simulink model "FFM_Punch"  (R2017a)
settings: Solver=ode3  StartTime=0.0  StopTime=timesteps  FixedStep=data.SIM.Ts  RelTol=1e-3  EnableMultiTasking=on
values from neighbouring files (symbols this model uses):
  data =     [dakota_config.mat]
  downshift_map = data.TCU.upshift.veh_spd_default    [Simulation_results.m]
  upshift_map = data.TCU.upshift.veh_spd_default    [Simulation_results.m]
undefined symbols (not defined in the file or in its folder): air_density, Cd, DiscIntNeverNeededParam, fr_crankshaft, fr_speed_values, g, i_FD, ICE, Low_Ratio, M_Eng_Max, M_Eng_Max_Max, M_Eng_Max_Rpm, mt2m_f, mu_Roll_C0, mu_Roll_C1, mu_Roll_C2, Mv, n_Idle_Eng, Overdrive_Ratio, Re, S_eff_drag, Ts
(part 11 of 15)

== system FFM_Punch/Driver Interface/Driver Model-_old/Driver Pedal Behaviour/Saturation Dynamic1 ==
  up : Inport
  u : Inport  Port=2
  lo : Inport  Port=3
  Data Type Duplicate : DataTypeDuplicate  DisableCoverage=on
  Data Type Propagation : S-Function  FunctionName=sfix_dtprop  Parameters=14,PropDataTypeMode,(getdatatypespecs(PropDataType,PropScaling,DblOver,0, 0, PropDataTypeMode, PropScalingMode)),IfRefDouble,IfRefSingle,IsSigned,NumBitsBase,NumBitsMult,NumBitsAdd,(sort(reshape(round(NumBitsAllowFinal), prod(size(NumBitsAllowFinal)),1))),PropScalingMode,ValuesUsedBestPrec,SlopeBase,SlopeMult,SlopeAdd,BiasBase,BiasMult,BiasAdd,DblOver  SFunctionDeploymentMode=off  EnableBusSupport=off  mask(Data Type Propagation){PropDataTypeMode=Inherit via propagation rule, PropDataType=fixdt(1, 16), IfRefDouble=double, IfRefSingle=single, IsSigned=IsSigned1, NumBitsBase=NumBits1, NumBitsMult=1, NumBitsAdd=0, NumBitsAllowFinal=1:128, PropScalingMode=Inherit via propagation rule, PropScaling=2^-10, ValuesUsedBestPrec=[5 -7], SlopeBase=Slope1, SlopeMult=1, SlopeAdd=0, BiasBase=Bias1, BiasMult=1, BiasAdd=0}
      mask prompts: PropDataTypeMode "Simulink:masks:x1PropagatedDataType_MP"; PropDataType "Simulink:masks:x11PropagatedDataTypeegFixdt116Fixdtsingle_MP"; IfRefDouble "Simulink:masks:x11IfAnyReferenceInputIsDoubleOutputIs_MP"; IfRefSingle "Simulink:masks:x12IfAnyReferenceInputIsSingleOutputIs_MP"; IsSigned "Simulink:masks:x13IsSigned_MP"; NumBitsBase "Simulink:masks:x141NumberofBitsBase_MP"; NumBitsMult "Simulink:masks:x142NumberofBitsMultiplicativeAdjustment_MP"; NumBitsAdd "Simulink:masks:x143NumberofBitsAdditiveAdjustment_MP"; NumBitsAllowFinal "Simulink:masks:x144NumberofBitsAllowableFinalValues_MP"; PropScalingMode "Simulink:masks:x2PropagatedScaling_MP"; PropScaling "Simulink:masks:x21PropagatedScalingSlopeEg29OrSlopeBiasEg1253_MP"; ValuesUsedBestPrec "Simulink:masks:x21ValuesUsedToDetermineBestPrecisionScaling_MP"; SlopeBase "Simulink:masks:x211SlopeBase_MP"; SlopeMult "Simulink:masks:x212SlopeMultiplicativeAdjustment_MP"; SlopeAdd "Simulink:masks:x213SlopeAdditiveAdjustment_MP"; BiasBase "Simulink:masks:x221BiasBase_MP"; BiasMult "Simulink:masks:x222BiasMultiplicativeAdjustment_MP"; BiasAdd "Simulink:masks:x223BiasAdditiveAdjustment_MP"
      mask help: Simulink:masks:DataTypePropagation_MD
      mask init:
      | DblOver = 0;
      mask TypeOptions PropDataTypeMode: Simulink:masks:SpecifyViaDialog | Simulink:masks:InheritViaPropagationRule
      mask Callback PropDataTypeMode: fixptdialog(gcbh)
      mask Callback PropDataType: fixptdialog(gcbh)
      mask TypeOptions IfRefDouble: Simulink:masks:double | Simulink:masks:single
      mask TypeOptions IfRefSingle: Simulink:masks:double | Simulink:masks:single
      mask TypeOptions IsSigned: Simulink:masks:IsSigned1 | Simulink:masks:IsSigned2 | Simulink:masks:IsSigned1OrIsSigned2 | Simulink:masks:TRUE | Simulink:masks:FALSE
      mask TypeOptions NumBitsBase: NumBits1 | NumBits2 | max([NumBits1 NumBits2]) | min([NumBits1 NumBits2]) | NumBits1+NumBits2
      mask TypeOptions PropScalingMode: Simulink:masks:SpecifyViaDialog | Simulink:masks:InheritViaPropagationRule | Simulink:masks:ObtainViaBestPrecision
      mask Callback PropScalingMode: fixptdialog(gcbh)
      mask TypeOptions SlopeBase: Slope1 | Slope2 | max([Slope1 Slope2]) | min([Slope1 Slope2]) | Slope1*Slope2 | Slope1/Slope2 | PosRange1 | PosRange2 | max([PosRange1 PosRange2]) | min([PosRange1 PosRange2]) | PosRange1*PosRange2 | PosRange1/PosRange2
      mask TypeOptions BiasBase: Bias1 | Bias2 | max([Bias1 Bias2]) | min([Bias1 Bias2]) | Bias1*Bias2 | Bias1/Bias2 | Bias1+Bias2 | Bias1-Bias2
      mask Display:
      | port_label('Input',1,'Ref1');
      | port_label('Input',2,'Ref2');
      | port_label('Input',3,'Prop');
  LowerRelop1 : RelationalOperator  DisableCoverage=on  Operator=>  OutDataTypeStr=boolean  RndMeth=Nearest
  Switch : Switch  Criteria=u2 ~= 0  OutDataTypeStr=Inherit: Inherit via back propagation  ZeroCross=off
  Switch2 : Switch  Criteria=u2 ~= 0  OutMin=OutMin  OutMax=OutMax  OutDataTypeStr=Inherit: Inherit via back propagation  ZeroCross=off
  UpperRelop : RelationalOperator  DisableCoverage=on  Operator=<  OutDataTypeStr=boolean  RndMeth=Nearest
  y : Outport  OutMin=OutMin  OutMax=OutMax
  wires:
  up/1 -> Switch2/1, LowerRelop1/2
  u/1 -> Data Type Propagation/2, Data Type Propagation/1, LowerRelop1/1, Switch/3, UpperRelop/1
  lo/1 -> Switch/1, UpperRelop/2
  Switch/1 -> Data Type Duplicate/2, Switch2/3, Data Type Propagation/3
  Switch2/1 -> Data Type Duplicate/1, y/1
  LowerRelop1/1 -> Switch2/2
  UpperRelop/1 -> Switch/2

== system FFM_Punch/Controller/F02_03_03_05_Raw_Gear_Target_Auto_Mode/F02_03_03_05_09_Final_Raw_Gear_Target_Auto_Mode/TurnOnDelay1/Rising_Edge_DetectChange1 ==
  b_Input : Inport  Tag=Controls_Lib  Description=Inp  OutDataTypeStr=boolean  Interpolate=off
  b_InitialValue : Inport  Tag=Controls_Lib  Description=Inp  Port=2  OutDataTypeStr=boolean  Interpolate=off
  Delay1 : Delay  Tag=Controls_Lib  Description=VariableDelay  DelayLength=DelayLength  DelayLengthUpperLimit=DelayLengthUpperLimit  InitialConditionSource=Input port  InitialCondition=InitialCondition  SampleTime=SampleTime  mask(Delay){DelayLengthSource=Dialog, DelayLength=1, DelayLengthUpperLimit=100, InitialConditionSource=Input port, InitialCondition=0.0, ExternalReset=None, PreventDirectFeedthrough=off, DiagnosticForOutOfRangeDelayLength=None, RemoveProtectionDelayLength=off, InputProcessing=Elements as channels (sample based), UseCircularBuffer=off, SampleTime=-1, StateName=, StateMustResolveToSignalObject=off, CodeGenStateStorageClass=Auto, CodeGenStateStorageTypeQualifier=}
      mask prompts: DelayLengthSource "Delay length source:"; DelayLength "Delay length:"; DelayLengthUpperLimit "Delay upper limit:"; InitialConditionSource "Initial condition source:"; InitialCondition "Initial condition:"; ExternalReset "External reset:"; PreventDirectFeedthrough "Prevent direct feedthrough by increasing delay length to lower limit"; DiagnosticForOutOfRangeDelayLength "Diagnostic for out-of-range delay length:"; RemoveProtectionDelayLength "Remove protection against out-of-range delay length in generated code"; InputProcessing "Input processing:"; UseCircularBuffer "Use circular buffer for state"; SampleTime "Sample time (-1 for inherited):"; StateName "State name:"; StateMustResolveToSignalObject "State name must resolve to Simulink signal object"; CodeGenStateStorageClass "Code generation storage class:"; CodeGenStateStorageTypeQualifier "Code generation storage type qualifier:"
      mask help: Delay input by a fixed or variable number of samples. The initial output of the delay block is specified by the external input x0.
      settings: InputPortMap=u0,p4
      mask Help: web([fileparts(which('Lib_discrete')) filesep 'hlp' filesep 'lib_Delay.html'], '-helpbrowser')
      mask TypeOptions DelayLengthSource: DelayLengthSource
      mask TypeOptions DelayLength: DelayLength
      mask TypeOptions DelayLengthUpperLimit: DelayLengthUpperLimit
      mask TypeOptions InitialConditionSource: InitialConditionSource
      mask TypeOptions InitialCondition: InitialCondition
      mask TypeOptions ExternalReset: ExternalReset
      mask TypeOptions PreventDirectFeedthrough: PreventDirectFeedthrough
      mask TypeOptions DiagnosticForOutOfRangeDelayLength: DiagnosticForOutOfRangeDelayLength
      mask TypeOptions RemoveProtectionDelayLength: RemoveProtectionDelayLength
      mask TypeOptions InputProcessing: InputProcessing
      mask TypeOptions UseCircularBuffer: UseCircularBuffer
      mask TypeOptions SampleTime: SampleTime
      mask TypeOptions StateName: StateName
      mask TypeOptions StateMustResolveToSignalObject: StateMustResolveToSignalObject
      mask TypeOptions CodeGenStateStorageClass: CodeGenStateStorageClass
      mask TypeOptions CodeGenStateStorageTypeQualifier: CodeGenStateStorageTypeQualifier
  Logic : Logic  Tag=Controls_Lib  Description=Logic  Operator=NOT  Inputs=Inputs  OutDataTypeStr=boolean  SampleTime=SampleTime  mask(Logic){Operator=NOT, Inputs=2, IconShape=rectangular, SampleTime=-1, AllPortsSameDT=on, OutDataTypeStr=boolean}
      mask prompts: Inputs "Number of input ports:"; IconShape "Icon shape:"; SampleTime "Sample time (-1 for inherited):"; AllPortsSameDT "Require all inputs and output to have the same data type"; OutDataTypeStr "Output data type:"
      mask help: Logical operators. For a single input, operators are applied across the input vector. For multiple inputs, operators are applied across the inputs.
      mask Help: web([fileparts(which('Lib_built')) filesep 'hlp' filesep 'lib_Logic' '.html'], '-helpbrowser')
      mask TypeOptions Operator: Operator
      mask TypeOptions Inputs: Inputs
      mask TypeOptions IconShape: IconShape
      mask TypeOptions SampleTime: SampleTime
      mask TypeOptions AllPortsSameDT: AllPortsSameDT
      mask TypeOptions OutDataTypeStr: OutDataTypeStr
  Logic1 : Logic  Tag=Controls_Lib  Description=Logic  Inputs=Inputs  OutDataTypeStr=boolean  SampleTime=SampleTime  mask(Logic){Operator=AND, Inputs=2, IconShape=rectangular, SampleTime=-1, AllPortsSameDT=on, OutDataTypeStr=boolean}
      mask prompts: Inputs "Number of input ports:"; IconShape "Icon shape:"; SampleTime "Sample time (-1 for inherited):"; AllPortsSameDT "Require all inputs and output to have the same data type"; OutDataTypeStr "Output data type:"
      mask help: Logical operators. For a single input, operators are applied across the input vector. For multiple inputs, operators are applied across the inputs.
      mask Help: web([fileparts(which('Lib_built')) filesep 'hlp' filesep 'lib_Logic' '.html'], '-helpbrowser')
      mask TypeOptions Operator: Operator
      mask TypeOptions Inputs: Inputs
      mask TypeOptions IconShape: IconShape
      mask TypeOptions SampleTime: SampleTime
      mask TypeOptions AllPortsSameDT: AllPortsSameDT
      mask TypeOptions OutDataTypeStr: OutDataTypeStr
  b_Output : Outport  Tag=Controls_Lib  OutDataTypeStr=boolean
  wires:
  Delay1/1 -> Logic/1
  Logic1/1 -> b_Output/1
  Logic/1 -> Logic1/2
  b_Input/1 -> Logic1/1, Delay1/1
  b_InitialValue/1 -> Delay1/2

== system FFM_Punch/Controller/F02_03_03_05_Raw_Gear_Target_Auto_Mode/F02_03_03_05_09_Final_Raw_Gear_Target_Auto_Mode/TurnOnDelay1/Timer ==
  note: Reset check
  Res : Inport  Tag=Controls_Lib_V1.0  OutDataTypeStr=boolean  Interpolate=off
  TT : Inport  Tag=Controls_Lib_V1.0  Port=2  OutDataTypeStr=single  Interpolate=off
  AddSub1 : Sum  Tag=Controls_Lib  Description=AddSub  Inputs=-+  CollapseDim=CollapseDim  AccumDataTypeStr=single  OutMin=OutMin  OutMax=OutMax  OutDataTypeStr=single  RndMeth=Nearest  SampleTime=SampleTime  InputSameDT=on  mask(AddSub){IconShape=rectangular, Inputs=-+, CollapseMode=All dimensions, CollapseDim=1, SampleTime=-1, InputSameDT=on, AccumDataTypeStr=single, OutMin=[], OutMax=[], OutDataTypeStr=single, LockScale=off, RndMeth=Nearest, SaturateOnIntegerOverflow=off}
      mask prompts: IconShape "Icon shape:"; Inputs "List of signs:"; CollapseMode "Sum over:"; CollapseDim "Dimension:"; SampleTime "Sample time (-1 for inherited):"; InputSameDT "Require all inputs to have the same data type"; AccumDataTypeStr "Accumulator data type:"; OutMin "Output minimum:"; OutMax "Output maximum:"; OutDataTypeStr "Output data type:"; LockScale "Lock data type settings against changes by the fixed-point tools"; RndMeth "Integer rounding mode:"; SaturateOnIntegerOverflow "Saturate on integer overflow"
      mask help:
      | Add or subtract inputs.  Specify one of the following:
      | a) string containing + or - for each input port, | for spacer between ports (e.g. ++|-|++)
      | b) scalar, >= 1, specifies the number of input ports to be summed.
      | When there is only one input port, add or subtract elements over all dimensions or one specified dimension
      mask Help: web([fileparts(which('Lib_built')) filesep 'hlp' filesep 'lib_AddSub' '.html'], '-helpbrowser')
      mask TypeOptions IconShape: IconShape
      mask TypeOptions Inputs: Inputs
      mask TypeOptions CollapseMode: CollapseMode
      mask TypeOptions CollapseDim: CollapseDim
      mask TypeOptions SampleTime: SampleTime
      mask TypeOptions InputSameDT: InputSameDT
      mask TypeOptions AccumDataTypeStr: AccumDataTypeStr
      mask TypeOptions OutMin: OutMin
      mask TypeOptions OutMax: OutMax
      mask TypeOptions OutDataTypeStr: OutDataTypeStr
      mask TypeOptions LockScale: LockScale
      mask TypeOptions RndMeth: RndMeth
      mask TypeOptions SaturateOnIntegerOverflow: SaturateOnIntegerOverflow
  Constant : Constant  Tag=Controls_Lib_V1.0  Value=Value  OutMin=OutMin  OutMax=OutMax  OutDataTypeStr=Inherit: Inherit via back propagation  SampleTime=SampleTime  FramePeriod=FramePeriod  mask(Constant){Value=0.5, VectorParams1D=on, SampleTime=-1, FramePeriod=inf, OutMin=[], OutMax=[], OutDataTypeStr=Inherit: Inherit via back propagation, LockScale=off}
      mask prompts: Value "Constant value:"; VectorParams1D "Interpret vector parameters as 1-D"; SampleTime "Sample time:"; FramePeriod "Frame period:"; OutMin "Output minimum:"; OutMax "Output maximum:"; OutDataTypeStr "Output data type:"; LockScale "Lock output data type setting against changes by the fixed-point tools"
      mask help: Output the constant specified by the 'Constant value' parameter.
      mask TypeOptions Value: Value
      mask TypeOptions VectorParams1D: VectorParams1D
      mask TypeOptions SampleTime: SampleTime
      mask TypeOptions FramePeriod: FramePeriod
      mask TypeOptions OutMin: OutMin
      mask TypeOptions OutMax: OutMax
      mask TypeOptions OutDataTypeStr: OutDataTypeStr
      mask TypeOptions LockScale: LockScale
      mask Display: disp(get_param(gcb,'Value'))
  Constant1 : Constant  Tag=Controls_Lib_V1.0  Value=Value  OutMin=OutMin  OutMax=OutMax  OutDataTypeStr=Inherit: Inherit via back propagation  SampleTime=SampleTime  FramePeriod=FramePeriod  mask(Constant){Value=0, VectorParams1D=on, SampleTime=-1, FramePeriod=inf, OutMin=[], OutMax=[], OutDataTypeStr=Inherit: Inherit via back propagation, LockScale=off}
      mask prompts: Value "Constant value:"; VectorParams1D "Interpret vector parameters as 1-D"; SampleTime "Sample time:"; FramePeriod "Frame period:"; OutMin "Output minimum:"; OutMax "Output maximum:"; OutDataTypeStr "Output data type:"; LockScale "Lock output data type setting against changes by the fixed-point tools"
      mask help: Output the constant specified by the 'Constant value' parameter.
      mask TypeOptions Value: Value
      mask TypeOptions VectorParams1D: VectorParams1D
      mask TypeOptions SampleTime: SampleTime
      mask TypeOptions FramePeriod: FramePeriod
      mask TypeOptions OutMin: OutMin
      mask TypeOptions OutMax: OutMax
      mask TypeOptions OutDataTypeStr: OutDataTypeStr
      mask TypeOptions LockScale: LockScale
      mask Display: disp(get_param(gcb,'Value'))
  Constant2 : Constant  Tag=Controls_Lib_V1.0  Value=Value  OutMin=OutMin  OutMax=OutMax  OutDataTypeStr=single  SampleTime=SampleTime  FramePeriod=FramePeriod  mask(Constant){Value=1, VectorParams1D=on, SampleTime=-1, FramePeriod=inf, OutMin=[], OutMax=[], OutDataTypeStr=single, LockScale=off}
      mask prompts: Value "Constant value:"; VectorParams1D "Interpret vector parameters as 1-D"; SampleTime "Sample time:"; FramePeriod "Frame period:"; OutMin "Output minimum:"; OutMax "Output maximum:"; OutDataTypeStr "Output data type:"; LockScale "Lock output data type setting against changes by the fixed-point tools"
      mask help: Output the constant specified by the 'Constant value' parameter.
      mask TypeOptions Value: Value
      mask TypeOptions VectorParams1D: VectorParams1D
      mask TypeOptions SampleTime: SampleTime
      mask TypeOptions FramePeriod: FramePeriod
      mask TypeOptions OutMin: OutMin
      mask TypeOptions OutMax: OutMax
      mask TypeOptions OutDataTypeStr: OutDataTypeStr
      mask TypeOptions LockScale: LockScale
      mask Display: disp(get_param(gcb,'Value'))
  Logical Operator : Logic  Operator=OR  AllPortsSameDT=off  OutDataTypeStr=boolean
  MulDiv : Product  Tag=Controls_Lib  Description=MulDiv  Inputs=**  CollapseDim=CollapseDim  OutMin=OutMin  OutMax=OutMax  OutDataTypeStr=single  SampleTime=SampleTime  InputSameDT=on  mask(MulDiv){Inputs=**, Multiplication=Element-wise(.*), CollapseMode=All dimensions, CollapseDim=1, SampleTime=-1, InputSameDT=on, OutMin=[], OutMax=[], OutDataTypeStr=single, LockScale=off, RndMeth=Floor, SaturateOnIntegerOverflow=off}
      mask prompts: Inputs "Number of inputs:"; CollapseMode "Multiply over:"; CollapseDim "Dimension:"; SampleTime "Sample time (-1 for inherited):"; InputSameDT "Require all inputs to have the same data type"; OutMin "Output minimum:"; OutMax "Output maximum:"; OutDataTypeStr "Output data type:"; LockScale "Lock output data type setting against changes by the fixed-point tools"; RndMeth "Integer rounding mode:"; SaturateOnIntegerOverflow "Saturate on integer overflow"
      mask help:
      | Multiply or divide inputs element-wise. Specify one of the following:
      |  a) * or / for each input port. For example, **/* performs the operation 'u1*u2/u3*u4'.
      |  b) scalar specifies the number of input ports to be multiplied.
      | If there is only one input port and the Multiplication parameter is set to Element-wise(.*), a single * or / collapses the input signal using the specified operation.
      mask Help: web([fileparts(which('Lib_built')) filesep 'hlp' filesep 'lib_MulDiv' '.html'], '-helpbrowser')
      mask TypeOptions Inputs: Inputs
      mask TypeOptions Multiplication: Multiplication
      mask TypeOptions CollapseMode: CollapseMode
      mask TypeOptions CollapseDim: CollapseDim
      mask TypeOptions SampleTime: SampleTime
      mask TypeOptions InputSameDT: InputSameDT
      mask TypeOptions OutMin: OutMin
      mask TypeOptions OutMax: OutMax
      mask TypeOptions OutDataTypeStr: OutDataTypeStr
      mask TypeOptions LockScale: LockScale
      mask TypeOptions RndMeth: RndMeth
      mask TypeOptions SaturateOnIntegerOverflow: SaturateOnIntegerOverflow
  MulDiv1 : Product  Tag=Controls_Lib  Description=MulDiv  Inputs=*/  CollapseDim=CollapseDim  OutMin=OutMin  OutMax=OutMax  OutDataTypeStr=single  SampleTime=SampleTime  InputSameDT=on  mask(MulDiv){Inputs=*/, Multiplication=Element-wise(.*), CollapseMode=All dimensions, CollapseDim=1, SampleTime=-1, InputSameDT=on, OutMin=[], OutMax=[], OutDataTypeStr=single, LockScale=off, RndMeth=Floor, SaturateOnIntegerOverflow=off}
      mask prompts: Inputs "Number of inputs:"; CollapseMode "Multiply over:"; CollapseDim "Dimension:"; SampleTime "Sample time (-1 for inherited):"; InputSameDT "Require all inputs to have the same data type"; OutMin "Output minimum:"; OutMax "Output maximum:"; OutDataTypeStr "Output data type:"; LockScale "Lock output data type setting against changes by the fixed-point tools"; RndMeth "Integer rounding mode:"; SaturateOnIntegerOverflow "Saturate on integer overflow"
      mask help:
      | Multiply or divide inputs element-wise. Specify one of the following:
      |  a) * or / for each input port. For example, **/* performs the operation 'u1*u2/u3*u4'.
      |  b) scalar specifies the number of input ports to be multiplied.
      | If there is only one input port and the Multiplication parameter is set to Element-wise(.*), a single * or / collapses the input signal using the specified operation.
      mask Help: web([fileparts(which('Lib_built')) filesep 'hlp' filesep 'lib_MulDiv' '.html'], '-helpbrowser')
      mask TypeOptions Inputs: Inputs
      mask TypeOptions Multiplication: Multiplication
      mask TypeOptions CollapseMode: CollapseMode
      mask TypeOptions CollapseDim: CollapseDim
      mask TypeOptions SampleTime: SampleTime
      mask TypeOptions InputSameDT: InputSameDT
      mask TypeOptions OutMin: OutMin
      mask TypeOptions OutMax: OutMax
      mask TypeOptions OutDataTypeStr: OutDataTypeStr
      mask TypeOptions LockScale: LockScale
      mask TypeOptions RndMeth: RndMeth
      mask TypeOptions SaturateOnIntegerOverflow: SaturateOnIntegerOverflow
  RelationalOperator : RelationalOperator  Tag=Controls_Lib_V1.0  Operator=>  OutDataTypeStr=boolean  SampleTime=SampleTime  RndMeth=Nearest  InputSameDT=on  mask(Relational operator){Operator=>, ZeroCross=on, SampleTime=-1, InputSameDT=on, OutDataTypeStr=boolean}
      mask prompts: Operator "Relational operator:"; ZeroCross "Enable zero-crossing detection"; SampleTime "Sample time (-1 for inherited):"; InputSameDT "Require all inputs to have the same data type"; OutDataTypeStr "Output data type:"
      mask help: Applies the selected relational operator to the inputs and outputs the result. The top (or left) input corresponds to the first operand.
      mask TypeOptions Operator: Operator
      mask TypeOptions ZeroCross: ZeroCross
      mask TypeOptions SampleTime: SampleTime
      mask TypeOptions InputSameDT: InputSameDT
      mask TypeOptions OutDataTypeStr: OutDataTypeStr
  RelationalOperator1 : RelationalOperator  Tag=Controls_Lib_V1.0  Operator=>  OutDataTypeStr=boolean  SampleTime=SampleTime  RndMeth=Nearest  InputSameDT=on  mask(Relational operator){Operator=>, ZeroCross=on, SampleTime=-1, InputSameDT=on, OutDataTypeStr=boolean}
      mask prompts: Operator "Relational operator:"; ZeroCross "Enable zero-crossing detection"; SampleTime "Sample time (-1 for inherited):"; InputSameDT "Require all inputs to have the same data type"; OutDataTypeStr "Output data type:"
      mask help: Applies the selected relational operator to the inputs and outputs the result. The top (or left) input corresponds to the first operand.
      mask TypeOptions Operator: Operator
      mask TypeOptions ZeroCross: ZeroCross
      mask TypeOptions SampleTime: SampleTime
      mask TypeOptions InputSameDT: InputSameDT
      mask TypeOptions OutDataTypeStr: OutDataTypeStr
  Switch : Switch  Tag=Controls_Lib  Description=Switch  Criteria=u2 ~= 0  Threshold=Threshold  OutMin=OutMin  OutMax=OutMax  OutDataTypeStr=Inherit: Inherit via back propagation  RndMeth=Zero  ZeroCross=off  SampleTime=SampleTime  InputSameDT=on  mask(Switch){Criteria=u2 ~= 0, Threshold=0.5, ZeroCross=off, SampleTime=-1, InputSameDT=on, OutMin=[], OutMax=[], OutDataTypeStr=Inherit: Inherit via back propagation, LockScale=off, RndMeth=Zero, SaturateOnIntegerOverflow=off, AllowDiffInputSizes=off}
      mask prompts: Criteria "Criteria for passing first input:"; ZeroCross "Enable zero-crossing detection"; SampleTime "Sample time (-1 for inherited):"; InputSameDT "Require all data port inputs to have the same data type"; OutMin "Output minimum:"; OutMax "Output maximum:"; OutDataTypeStr "Output data type:"; LockScale "Lock output data type setting against changes by the fixed-point tools"; RndMeth "Integer rounding mode:"; SaturateOnIntegerOverflow "Saturate on integer overflow"; AllowDiffInputSizes "Allow different data input sizes (Results in variable-size output signal)"
      mask help: Pass through input 1 when input 2 is greater than 0 otherwise, pass through input 3. The inputs are numbered top to bottom (or left to right). The input 1 pass-through criteria are input 2 greater than or equal, greater than, or not equal to the threshold. The first and third input ports are data ports, and the second input port is the control port. The control port signal should always be a boolean signal.
      mask Help: web([fileparts(which('Lib_built')) filesep 'hlp' filesep 'lib_Switch' '.html'], '-helpbrowser')
      mask TypeOptions Criteria: Criteria
      mask TypeOptions Threshold: Threshold
      mask TypeOptions ZeroCross: ZeroCross
      mask TypeOptions SampleTime: SampleTime
      mask TypeOptions InputSameDT: InputSameDT
      mask TypeOptions OutMin: OutMin
      mask TypeOptions OutMax: OutMax
      mask TypeOptions OutDataTypeStr: OutDataTypeStr
      mask TypeOptions LockScale: LockScale
      mask TypeOptions RndMeth: RndMeth
      mask TypeOptions SaturateOnIntegerOverflow: SaturateOnIntegerOverflow
      mask TypeOptions AllowDiffInputSizes: AllowDiffInputSizes
  Switch1 : Switch  Tag=Controls_Lib  Description=Switch  Criteria=u2 ~= 0  Threshold=Threshold  OutMin=OutMin  OutMax=OutMax  OutDataTypeStr=Inherit: Inherit via back propagation  RndMeth=Zero  ZeroCross=off  SampleTime=SampleTime  InputSameDT=on  mask(Switch){Criteria=u2 ~= 0, Threshold=0.5, ZeroCross=off, SampleTime=-1, InputSameDT=on, OutMin=[], OutMax=[], OutDataTypeStr=Inherit: Inherit via back propagation, LockScale=off, RndMeth=Zero, SaturateOnIntegerOverflow=off, AllowDiffInputSizes=off}
      mask prompts: Criteria "Criteria for passing first input:"; ZeroCross "Enable zero-crossing detection"; SampleTime "Sample time (-1 for inherited):"; InputSameDT "Require all data port inputs to have the same data type"; OutMin "Output minimum:"; OutMax "Output maximum:"; OutDataTypeStr "Output data type:"; LockScale "Lock output data type setting against changes by the fixed-point tools"; RndMeth "Integer rounding mode:"; SaturateOnIntegerOverflow "Saturate on integer overflow"; AllowDiffInputSizes "Allow different data input sizes (Results in variable-size output signal)"
      mask help: Pass through input 1 when input 2 is greater than 0 otherwise, pass through input 3. The inputs are numbered top to bottom (or left to right). The input 1 pass-through criteria are input 2 greater than or equal, greater than, or not equal to the threshold. The first and third input ports are data ports, and the second input port is the control port. The control port signal should always be a boolean signal.
      mask Help: web([fileparts(which('Lib_built')) filesep 'hlp' filesep 'lib_Switch' '.html'], '-helpbrowser')
      mask TypeOptions Criteria: Criteria
      mask TypeOptions Threshold: Threshold
      mask TypeOptions ZeroCross: ZeroCross
      mask TypeOptions SampleTime: SampleTime
      mask TypeOptions InputSameDT: InputSameDT
      mask TypeOptions OutMin: OutMin
      mask TypeOptions OutMax: OutMax
      mask TypeOptions OutDataTypeStr: OutDataTypeStr
      mask TypeOptions LockScale: LockScale
      mask TypeOptions RndMeth: RndMeth
      mask TypeOptions SaturateOnIntegerOverflow: SaturateOnIntegerOverflow
      mask TypeOptions AllowDiffInputSizes: AllowDiffInputSizes
  TsInverse : SampleTimeMath  TsampMathOp=1/Ts Only  weightValue=weightValue  OutDataTypeStr=Inherit: Inherit via back propagation  mask(Sample time block){TsampMathOp=1/Ts Only, weightValue=1, TsampMathImp=Online Calculations, OutDataTypeStr=Inherit: Inherit via back propagation, RndMeth=Floor, SaturateOnIntegerOverflow=off}
      mask prompts: TsampMathOp "Operation:"; weightValue "Weight value:"; TsampMathImp "Implement using:"; OutDataTypeStr "Output data type:"; RndMeth "Integer rounding mode:"; SaturateOnIntegerOverflow "Saturate on integer overflow"
      mask help: 1 divided by the Sample time of the input signal
      mask Help: web([fileparts(which('Lib_built')) filesep 'hlp' filesep 'lib_TsInv' '.html'], '-helpbrowser')
      mask TypeOptions TsampMathOp: TsampMathOp
      mask TypeOptions weightValue: weightValue
      mask TypeOptions TsampMathImp: TsampMathImp
      mask TypeOptions OutDataTypeStr: OutDataTypeStr
      mask TypeOptions RndMeth: RndMeth
      mask TypeOptions SaturateOnIntegerOverflow: SaturateOnIntegerOverflow
  UnitDelay : UnitDelay  Tag=Controls_Lib  Description=UnitDelay  InitialCondition=X0  SampleTime=SampleTime  mask(Unit delay){X0=0, InputProcessing=Elements as channels (sample based), SampleTime=-1, StateIdentifier=, StateMustResolveToSignalObject=off, RTWStateStorageClass=Auto, RTWStateStorageTypeQualifier=}
      mask prompts: X0 "Initial conditions:"; InputProcessing "Input processing:"; SampleTime "Sample time (-1 for inherited):"; StateIdentifier "State name:"; StateMustResolveToSignalObject "State name must resolve to Simulink signal object"; RTWStateStorageClass "Code generation storage class:"; RTWStateStorageTypeQualifier "Code generation storage type qualifier:"
      mask help: Delays input signal one sample period
      settings: AttributesFormatString=Init_con=%<X0>
      mask TypeOptions X0: X0
      mask TypeOptions InputProcessing: InputProcessing
      mask TypeOptions SampleTime: SampleTime
      mask TypeOptions StateIdentifier: StateIdentifier
      mask TypeOptions StateMustResolveToSignalObject: StateMustResolveToSignalObject
      mask TypeOptions RTWStateStorageClass: RTWStateStorageClass
      mask TypeOptions RTWStateStorageTypeQualifier: RTWStateStorageTypeQualifier
  falling_edge : Subsystem  StopFcn=%tagged  TreatAsAtomicUnit=on  mask(Falling edge detection){}
      mask help:
      | Falling edge detection for a logic signal.
      | When a falling edge on the input signal is detected, the output switches to 1 during one time step.
      settings: RTWSystemCode=Nonreusable function
      mask Display: plot(0,0,100,100, [20 50 50 80], [90 90 10 10], [40 50 60], [55 45 55] )
  Busy : Outport  Tag=Controls_Lib_V1.0  OutDataTypeStr=boolean  InitialOutput=0
  TL : Outport  Tag=Controls_Lib_V1.0  Port=2  OutDataTypeStr=single  InitialOutput=0
  wires:
  [Ts] -> MulDiv/1
  MulDiv1/1 -> [Ts]
  TsInverse/1 -> MulDiv1/2
  Constant2/1 -> MulDiv1/1
  AddSub1/1 -> Switch/3
  [Ts] -> AddSub1/1
  Switch1/1 -> TsInverse/1, AddSub1/2, TL/1
  MulDiv/1 -> RelationalOperator/2, RelationalOperator1/1
  Switch/1 -> UnitDelay/1
  TT/1 -> Switch/1
  UnitDelay/1 -> RelationalOperator/1, RelationalOperator1/2, Switch1/3
  Constant/1 -> MulDiv/2
  RelationalOperator/1 -> falling_edge/1(Signal), Busy/1
  RelationalOperator1/1 -> Switch1/2
  Constant1/1 -> Switch1/1
  Logical Operator/1 -> Switch/2
  Res/1 -> Logical Operator/2
  falling_edge/1(Out) -> Logical Operator/1

== system FFM_Punch/Controller/F02_03_03_05_Raw_Gear_Target_Auto_Mode/F02_03_03_05_09_Final_Raw_Gear_Target_Auto_Mode/TurnOnDelay2/Rising_Edge_DetectChange1 ==
  b_Input : Inport  Tag=Controls_Lib  Description=Inp  OutDataTypeStr=boolean  Interpolate=off
  b_InitialValue : Inport  Tag=Controls_Lib  Description=Inp  Port=2  OutDataTypeStr=boolean  Interpolate=off
  Delay1 : Delay  Tag=Controls_Lib  Description=VariableDelay  DelayLength=DelayLength  DelayLengthUpperLimit=DelayLengthUpperLimit  InitialConditionSource=Input port  InitialCondition=InitialCondition  SampleTime=SampleTime  mask(Delay){DelayLengthSource=Dialog, DelayLength=1, DelayLengthUpperLimit=100, InitialConditionSource=Input port, InitialCondition=0.0, ExternalReset=None, PreventDirectFeedthrough=off, DiagnosticForOutOfRangeDelayLength=None, RemoveProtectionDelayLength=off, InputProcessing=Elements as channels (sample based), UseCircularBuffer=off, SampleTime=-1, StateName=, StateMustResolveToSignalObject=off, CodeGenStateStorageClass=Auto, CodeGenStateStorageTypeQualifier=}
      mask prompts: DelayLengthSource "Delay length source:"; DelayLength "Delay length:"; DelayLengthUpperLimit "Delay upper limit:"; InitialConditionSource "Initial condition source:"; InitialCondition "Initial condition:"; ExternalReset "External reset:"; PreventDirectFeedthrough "Prevent direct feedthrough by increasing delay length to lower limit"; DiagnosticForOutOfRangeDelayLength "Diagnostic for out-of-range delay length:"; RemoveProtectionDelayLength "Remove protection against out-of-range delay length in generated code"; InputProcessing "Input processing:"; UseCircularBuffer "Use circular buffer for state"; SampleTime "Sample time (-1 for inherited):"; StateName "State name:"; StateMustResolveToSignalObject "State name must resolve to Simulink signal object"; CodeGenStateStorageClass "Code generation storage class:"; CodeGenStateStorageTypeQualifier "Code generation storage type qualifier:"
      mask help: Delay input by a fixed or variable number of samples. The initial output of the delay block is specified by the external input x0.
      settings: InputPortMap=u0,p4
      mask Help: web([fileparts(which('Lib_discrete')) filesep 'hlp' filesep 'lib_Delay.html'], '-helpbrowser')
      mask TypeOptions DelayLengthSource: DelayLengthSource
      mask TypeOptions DelayLength: DelayLength
      mask TypeOptions DelayLengthUpperLimit: DelayLengthUpperLimit
      mask TypeOptions InitialConditionSource: InitialConditionSource
      mask TypeOptions InitialCondition: InitialCondition
      mask TypeOptions ExternalReset: ExternalReset
      mask TypeOptions PreventDirectFeedthrough: PreventDirectFeedthrough
      mask TypeOptions DiagnosticForOutOfRangeDelayLength: DiagnosticForOutOfRangeDelayLength
      mask TypeOptions RemoveProtectionDelayLength: RemoveProtectionDelayLength
      mask TypeOptions InputProcessing: InputProcessing
      mask TypeOptions UseCircularBuffer: UseCircularBuffer
      mask TypeOptions SampleTime: SampleTime
      mask TypeOptions StateName: StateName
      mask TypeOptions StateMustResolveToSignalObject: StateMustResolveToSignalObject
      mask TypeOptions CodeGenStateStorageClass: CodeGenStateStorageClass
      mask TypeOptions CodeGenStateStorageTypeQualifier: CodeGenStateStorageTypeQualifier
  Logic : Logic  Tag=Controls_Lib  Description=Logic  Operator=NOT  Inputs=Inputs  OutDataTypeStr=boolean  SampleTime=SampleTime  mask(Logic){Operator=NOT, Inputs=2, IconShape=rectangular, SampleTime=-1, AllPortsSameDT=on, OutDataTypeStr=boolean}
      mask prompts: Inputs "Number of input ports:"; IconShape "Icon shape:"; SampleTime "Sample time (-1 for inherited):"; AllPortsSameDT "Require all inputs and output to have the same data type"; OutDataTypeStr "Output data type:"
      mask help: Logical operators. For a single input, operators are applied across the input vector. For multiple inputs, operators are applied across the inputs.
      mask Help: web([fileparts(which('Lib_built')) filesep 'hlp' filesep 'lib_Logic' '.html'], '-helpbrowser')
      mask TypeOptions Operator: Operator
      mask TypeOptions Inputs: Inputs
      mask TypeOptions IconShape: IconShape
      mask TypeOptions SampleTime: SampleTime
      mask TypeOptions AllPortsSameDT: AllPortsSameDT
      mask TypeOptions OutDataTypeStr: OutDataTypeStr
  Logic1 : Logic  Tag=Controls_Lib  Description=Logic  Inputs=Inputs  OutDataTypeStr=boolean  SampleTime=SampleTime  mask(Logic){Operator=AND, Inputs=2, IconShape=rectangular, SampleTime=-1, AllPortsSameDT=on, OutDataTypeStr=boolean}
      mask prompts: Inputs "Number of input ports:"; IconShape "Icon shape:"; SampleTime "Sample time (-1 for inherited):"; AllPortsSameDT "Require all inputs and output to have the same data type"; OutDataTypeStr "Output data type:"
      mask help: Logical operators. For a single input, operators are applied across the input vector. For multiple inputs, operators are applied across the inputs.
      mask Help: web([fileparts(which('Lib_built')) filesep 'hlp' filesep 'lib_Logic' '.html'], '-helpbrowser')
      mask TypeOptions Operator: Operator
      mask TypeOptions Inputs: Inputs
      mask TypeOptions IconShape: IconShape
      mask TypeOptions SampleTime: SampleTime
      mask TypeOptions AllPortsSameDT: AllPortsSameDT
      mask TypeOptions OutDataTypeStr: OutDataTypeStr
  b_Output : Outport  Tag=Controls_Lib  OutDataTypeStr=boolean
  wires:
  Delay1/1 -> Logic/1
  Logic1/1 -> b_Output/1
  Logic/1 -> Logic1/2
  b_Input/1 -> Logic1/1, Delay1/1
  b_InitialValue/1 -> Delay1/2
